simulink model "Nealinearni_realni_v2"  (R2023b)
settings: Solver=ode23t  StartTime=0.0  StopTime=stepp.sim_time  RelTol=1e-3
undefined symbols (not defined in the file or in its folder): boost, ccm_m_op, Ci, dcm_op, dcm_separate_tfs, G_sys_ccm, Ipv0, m0_ccm, pv, Ramp, Ru, sim_op, stepp
libraries: spsSeriesRLCBranchLib x6, spsCurrentMeasurementLib x3, spsVoltageMeasurementLib x3, spsBistableLib x2, dspstat3 x2, dspfdesign x1, spsDiodeLib x1, spsControlledCurrentSourceLib x1, spsIdealSwitchLib x1, simulink_extras x1, simulink x1, sps_lib x1
settings Model: Creator=teo  LastModifiedBy=teo
settings HardwareCC: ProdBitPerLong=64  ProdHWDeviceType=AMD->x86-64 (Linux 64)

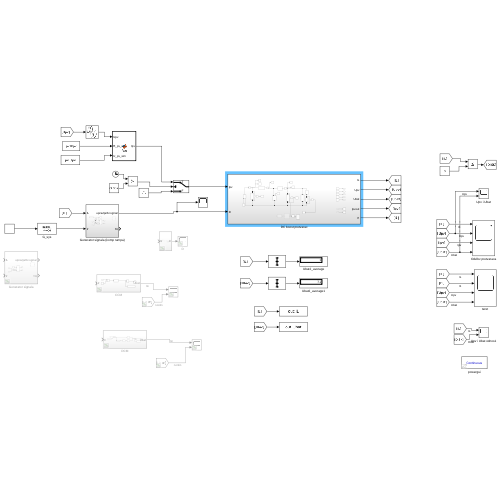
[thumbnail: Simulink's stored preview of the top-level diagram]
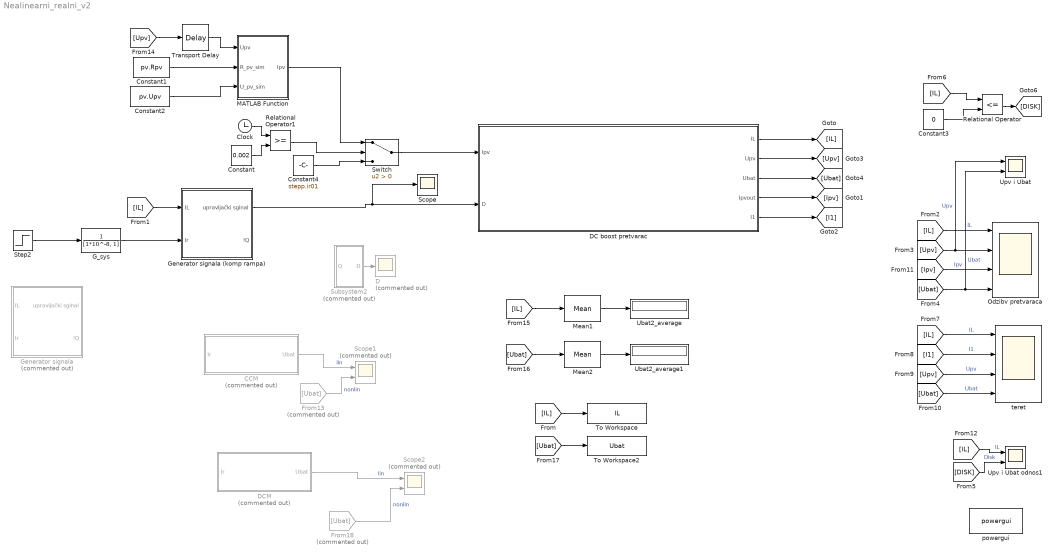
== system Nealinearni_realni_v2 ==
  CCM : Subsystem  Commented=on
  Clock : Clock
  Constant : Constant  Value=0.002
  Constant1 : Constant  Value=pv.Rpv
  Constant2 : Constant  Value=pv.Upv
  Constant3 : Constant  Value=0
  Constant4 : Constant  Value=stepp.ir01
  D : Scope  Commented=on
  DC boost pretvarac : Subsystem
  DCM : Subsystem  Commented=on
  From13 : From  Commented=on  GotoTag=Ubat
  From18 : From  Commented=on  GotoTag=Ubat
  G_sys : TransferFcn  Numerator=1  Denominator=[1*10^-8, 1]
  Generator signala : Subsystem  Commented=on
  Generator signala (komp rampa) : Subsystem
  MATLAB Function : MATLAB Function  TreatAsAtomicUnit=on
  Mean1 : dspstat3/Mean  run=off  InputProcessing=Columns as channels (frame based)  reset_popup=None  directionMode=Entire input  dimension=1  roiEnable=off  roiType=Rectangles  roiPortion=Entire ROI  roiOutput=Individual statistics for each ROI  roiFlag=off  roundingMode=Floor  overflowMode=off  outputDataTypeStr=Inherit: Same as accumulator  outputMin=[]  outputMax=[]  outputLastDataTypeStr=Inherit: Same as accumulator
  Mean2 : dspstat3/Mean  run=off  InputProcessing=Columns as channels (frame based)  reset_popup=None  directionMode=Entire input  dimension=1  roiEnable=off  roiType=Rectangles  roiPortion=Entire ROI  roiOutput=Individual statistics for each ROI  roiFlag=off  roundingMode=Floor  overflowMode=off  outputDataTypeStr=Inherit: Same as accumulator  outputMin=[]  outputMax=[]  outputLastDataTypeStr=Inherit: Same as accumulator
  Odzibv pretvaraca : Scope  NumInputPorts=4
  Relational Operator : RelationalOperator  Operator=<=  OutDataTypeStr=boolean  RndMeth=Simplest  InputSameDT=off
  Relational Operator1 : RelationalOperator  OutDataTypeStr=boolean  RndMeth=Simplest  InputSameDT=off
  Scope : Scope
  Scope1 : Scope  Commented=on  NumInputPorts=2
  Scope2 : Scope  Commented=on  NumInputPorts=2
  Step2 : Step  Time=stepp.step_time  Before=stepp.ir01  After=stepp.ir02  SampleTime=0
  Subsystem2 : Subsystem  Commented=on
  Switch : Switch  Criteria=u2 > Threshold  SaturateOnIntegerOverflow=off  InputSameDT=off
  To Workspace : ToWorkspace  VariableName=IL  SaveFormat=Timeseries  SampleTime=1e-6
  To Workspace2 : ToWorkspace  VariableName=Ubat  SaveFormat=Timeseries  SampleTime=1e-6
  Transport Delay : TransportDelay  DelayTime=0.001  BufferSize=4024
  Ubat2_average : Display
  Ubat2_average1 : Display
  Upv i Ubat : Scope  NumInputPorts=2
  Upv i Ubat odnos1 : Scope  NumInputPorts=2
  powergui : sps_lib/powergui  Priority=1  SimulationMode=Continuous  SampleTime=50e-6  frequency=60  Iterations=50  frequencyindice=0  Pbase=100e6  ErrMax=1e-4  UnitsV=kV  UnitsW=MW  buscounter=0  FunctionMessages=off  echomessages=off  EnableUseOfTLC=off  CurrentSourceSwitches=off  DisableSnubberDevices=off  DisableRonSwitches=off  DisableVfSwitches=off  DisplayEquations=off  AutomaticDiscreteSolvers=off  SolverType=Tustin/Backward Euler (TBE)  Interpol=off  ExternalGateDelay=off  methode=off  Ts=100  x0status=blocks  SPID=on  SwTol=0  HookPort=off  NonlinearTolerance=1e-4  nMaxIteration=100  ContinueOnMaxIteration=off  RestoreLinks=warning  ResistiveCurrentMeasurement=off  Frange=[0:2:500]  Ylog=off  Xlog=on  ShowGrid=off  save=off  variable=ZData  structure=0  ZoomFFT=off  StartTime=0.0  cycles=1  DisplayStyle=1  fundamental=60  FreqAxis=off  MaxFrequency=1000  frequencyindicesteady=1  RmsSteady=1  display=off
  teret : Scope  NumInputPorts=4
  wires:
  [IL] -> Odzibv pretvaraca/1  "IL"
  [Upv] -> Upv i Ubat/1, Odzibv pretvaraca/2  "Upv"
  [IL] -> teret/1  "IL"
  [I1] -> teret/2  "I1"
  [Upv] -> teret/3  "Upv"
  [IL] -> Upv i Ubat odnos1/1  "IL"
  [DISK] -> Upv i Ubat odnos1/2  "Disk"
  [Ipv] -> Odzibv pretvaraca/3  "Ipv"
  [IL] -> Relational Operator/1
  Relational Operator/1 -> [DISK]
  Constant3/1 -> Relational Operator/2
  [Ubat] -> Upv i Ubat/2, Odzibv pretvaraca/4  "Ubat"
  [Ubat] -> teret/4  "Ubat"
  DC boost pretvarac/2(Upv) -> [Upv]
  DC boost pretvarac/1(IL) -> [IL]
  DC boost pretvarac/3(Ubat) -> [Ubat]
  DC boost pretvarac/4(Ipvout) -> [Ipv]
  DC boost pretvarac/5(I1) -> [I1]
  [IL] -> Mean1/1
  Mean1/1 -> Ubat2_average/1
  [Ubat] -> Mean2/1
  Mean2/1 -> Ubat2_average1/1
  [IL] -> To Workspace/1
  [Ubat] -> To Workspace2/1
  Subsystem2/1(D) -> D/1
  Constant1/1 -> MATLAB Function/2(R_pv_sim)
  Constant2/1 -> MATLAB Function/3(U_pv_sim)
  [Upv] -> Transport Delay/1
  Transport Delay/1 -> MATLAB Function/1(Upv)
  Switch/1 -> DC boost pretvarac/1(Ipv)
  Clock/1 -> Relational Operator1/1
  Constant/1 -> Relational Operator1/2
  Relational Operator1/1 -> Switch/2
  Constant4/1 -> Switch/3
  MATLAB Function/1(Ipv) -> Switch/1
  CCM/1(Ubat) -> Scope1/1  "lin"
  From13/1 -> Scope1/2  "nonlin"
  DCM/1(Ubat) -> Scope2/1  "lin"
  From18/1 -> Scope2/2  "nonlin"
  [IL] -> Generator signala (komp rampa)/1(IL)
  Generator signala (komp rampa)/1(upravljački sginal) -> Scope/1, DC boost pretvarac/2(D)
  Step2/1 -> G_sys/1
  G_sys/1 -> Generator signala (komp rampa)/2(Ir)

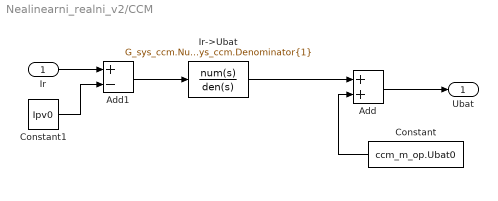
== system Nealinearni_realni_v2/CCM ==
  Ir : Inport
  Add : Sum
  Add1 : Sum  Inputs=+-
  Constant : Constant  Value=ccm_m_op.Ubat0
  Constant1 : Constant  Value=Ipv0
  Ir->Ubat : TransferFcn  Numerator=G_sys_ccm.Numerator{1}  Denominator=G_sys_ccm.Denominator{1}
  Ubat : Outport
  wires:
  Ir/1 -> Add1/1
  Constant1/1 -> Add1/2
  Add1/1 -> Ir->Ubat/1
  Add/1 -> Ubat/1
  Constant/1 -> Add/2
  Ir->Ubat/1 -> Add/1

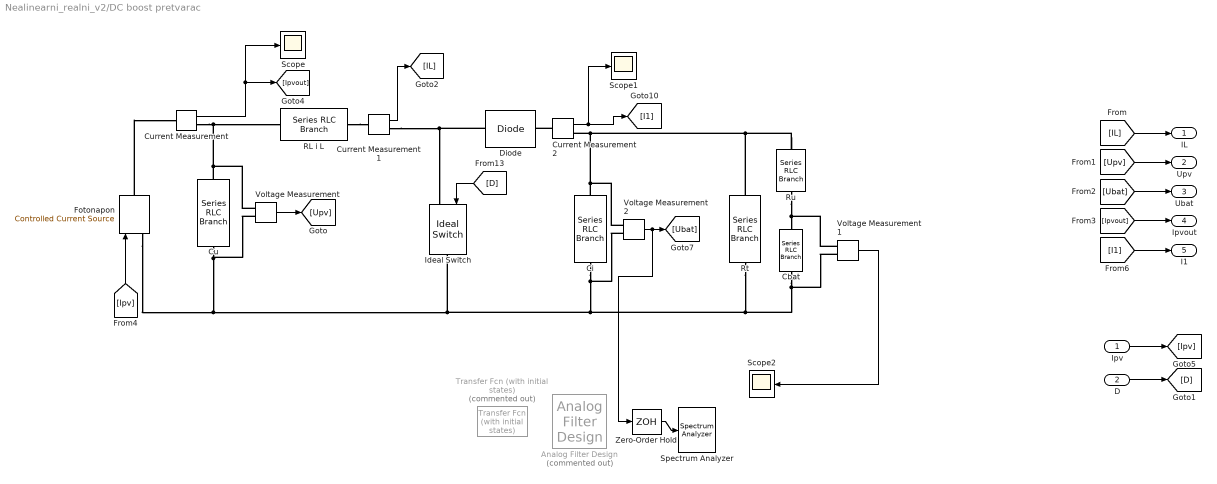
== system Nealinearni_realni_v2/DC boost pretvarac ==
  Ipv : Inport
  D : Inport  Port=2
  Analog Filter Design : dspfdesign/Analog Filter Design  Commented=on  method=Elliptic  filttype=Lowpass  N=8  Wlo=2*pi*boost.f  Whi=80  Rp=1  Rs=100
  Cbat : spsSeriesRLCBranchLib/Series RLC Branch  LConnTagsString=__new0  RConnTagsString=__new0  BranchType=C  Resistance=Ru  Inductance=1e-3  SetiL0=off  InitialCurrent=0  Capacitance=boost.Cbat  Setx0=on  InitialVoltage=sim_op.Ubat0  Measurements=None
  Ci : spsSeriesRLCBranchLib/Series RLC Branch  LConnTagsString=__new0  RConnTagsString=__new0  BranchType=C  Resistance=0.001  Inductance=1e-3  SetiL0=off  InitialCurrent=0  Capacitance=boost.Ci  Setx0=on  InitialVoltage=dcm_op.Ubat0  Measurements=None
  Cu : spsSeriesRLCBranchLib/Series RLC Branch  LConnTagsString=__new0  RConnTagsString=__new0  BranchType=C  Resistance=0.001  Inductance=1e-3  SetiL0=off  InitialCurrent=0  Capacitance=boost.Cu  Setx0=on  InitialVoltage=sim_op.Upv0  Measurements=None
  Current Measurement : spsCurrentMeasurementLib/Current Measurement  PhasorSimulation=off  OutputType=Complex  PSBequivalent=0
  Current Measurement1 : spsCurrentMeasurementLib/Current Measurement  PhasorSimulation=off  OutputType=Complex  PSBequivalent=0
  Current Measurement2 : spsCurrentMeasurementLib/Current Measurement  PhasorSimulation=off  OutputType=Complex  PSBequivalent=0
  Diode : spsDiodeLib/Diode  Ron=0  Lon=0  Vf=0  IC=0  UseSnubber=0  Rs=0  Cs=0  Measurements=off
  Fotonapon : spsControlledCurrentSourceLib/Controlled Current Source  Initialize=on  Source_Type=DC  Amplitude=0  Phase=0  Frequency=0  Measurements=None
  Ideal Switch : spsIdealSwitchLib/Ideal Switch  Ron=0  Lon=0  IC=0  Rs=0  Cs=0  Measurements=off
  RL i L : spsSeriesRLCBranchLib/Series RLC Branch  LConnTagsString=__new0  RConnTagsString=__new0  BranchType=RL  Resistance=boost.RL  Inductance=boost.L  SetiL0=off  InitialCurrent=Ipv0  Capacitance=1e-6  Setx0=off  InitialVoltage=0  Measurements=None
  Rt : spsSeriesRLCBranchLib/Series RLC Branch  LConnTagsString=__new0  RConnTagsString=__new0  BranchType=R  Resistance=boost.Rt  Inductance=1e-3  SetiL0=off  InitialCurrent=0  Capacitance=Ci  Setx0=off  InitialVoltage=0  Measurements=None
  Ru : spsSeriesRLCBranchLib/Series RLC Branch  LConnTagsString=__new0  RConnTagsString=__new0  BranchType=R  Resistance=boost.Ru  Inductance=1e-3  SetiL0=off  InitialCurrent=0  Capacitance=Ci  Setx0=on  InitialVoltage=Ubat0_ccm  Measurements=None
  Scope : Scope
  Scope1 : Scope
  Scope2 : Scope
  Spectrum Analyzer : SpectrumAnalyzer  WindowPosition=[1.000000,1.000000,1920.000000,1048.000000,]  Visible=on  ScopeFrameLocation=window  Method=Welch  PlotAsTwoSidedSpectrum=off  Span=150000  CenterFrequency=75000  StartFrequency=0  StopFrequency=150000  AveragingMethod=Exponential  ForgettingFactor=1  YLimits=[-161.71301101,85.74204889]  ExpandToolstrip=on  SelectedToolstripTab=spectrumAnalyzerToolstrip.measurementsTab
  Transfer Fcn (with initial states) : simulink_extras/Additional Linear/Transfer Fcn (with initial states)  Commented=on  N=[1]  D=[boost.Tmfc, 1]  X0=.5
  Voltage Measurement : spsVoltageMeasurementLib/Voltage Measurement  PhasorSimulation=off  OutputType=Complex  PSBequivalent=0
  Voltage Measurement1 : spsVoltageMeasurementLib/Voltage Measurement  PhasorSimulation=off  OutputType=Complex  PSBequivalent=0
  Voltage Measurement2 : spsVoltageMeasurementLib/Voltage Measurement  PhasorSimulation=off  OutputType=Complex  PSBequivalent=0
  Zero-Order Hold : ZeroOrderHold  SampleTime=1/(3*boost.f)
  IL : Outport
  Upv : Outport  Port=2
  Ubat : Outport  Port=3
  Ipvout : Outport  Port=4
  I1 : Outport  Port=5
  wires:
  Current Measurement1/1 -> [IL]
  Voltage Measurement/1 -> [Upv]
  [D] -> Ideal Switch/1
  [Ipv] -> Fotonapon/1
  D/1 -> [D]
  Ipv/1 -> [Ipv]
  [IL] -> IL/1
  [Upv] -> Upv/1
  [Ubat] -> Ubat/1
  Current Measurement/1 -> Scope/1, [Ipvout]
  [Ipvout] -> Ipvout/1
  Current Measurement2/1 -> Scope1/1, [I1]
  [I1] -> I1/1
  Voltage Measurement2/1 -> Zero-Order Hold/1, [Ubat]
  Voltage Measurement1/1 -> Scope2/1
  Zero-Order Hold/1 -> Spectrum Analyzer/1
  connections:
  Current Measurement/RConn1 -- Voltage Measurement/LConn1 -- Cu/LConn1 -- RL i L/LConn1
  RL i L/RConn1 -- Current Measurement1/LConn1
  Diode/LConn1 -- Ideal Switch/LConn1 -- Current Measurement1/RConn1
  Current Measurement2/LConn1 -- Diode/RConn1
  Ci/RConn1 -- Voltage Measurement2/LConn2 -- Voltage Measurement1/LConn2 -- Cbat/RConn1 -- Rt/RConn1 -- Voltage Measurement/LConn2 -- Cu/RConn1 -- Fotonapon/LConn1 -- Ideal Switch/RConn1
  Fotonapon/RConn1 -- Current Measurement/LConn1
  Ci/LConn1 -- Voltage Measurement2/LConn1 -- Rt/LConn1 -- Ru/LConn1 -- Current Measurement2/RConn1
  Ru/RConn1 -- Voltage Measurement1/LConn1 -- Cbat/LConn1

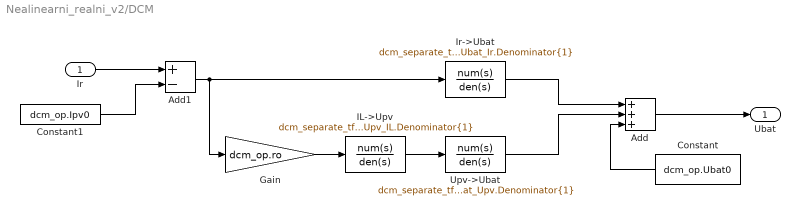
== system Nealinearni_realni_v2/DCM ==
  Ir : Inport
  Add : Sum  Inputs=+++
  Add1 : Sum  Inputs=+-
  Constant : Constant  Value=dcm_op.Ubat0
  Constant1 : Constant  Value=dcm_op.Ipv0
  Gain : Gain  Gain=dcm_op.ro
  IL->Upv : TransferFcn  Numerator=dcm_separate_tfs.G_Upv_IL.Numerator{1}  Denominator=dcm_separate_tfs.G_Upv_IL.Denominator{1}
  Ir->Ubat : TransferFcn  Numerator=dcm_separate_tfs.G_Ubat_Ir.Numerator{1}  Denominator=dcm_separate_tfs.G_Ubat_Ir.Denominator{1}
  Upv->Ubat : TransferFcn  Numerator=dcm_separate_tfs.G_Ubat_Upv.Numerator{1}  Denominator=dcm_separate_tfs.G_Ubat_Upv.Denominator{1}
  Ubat : Outport
  wires:
  Ir/1 -> Add1/1
  Add/1 -> Ubat/1
  Ir->Ubat/1 -> Add/1
  Constant1/1 -> Add1/2
  Upv->Ubat/1 -> Add/2
  Constant/1 -> Add/3
  IL->Upv/1 -> Upv->Ubat/1
  Add1/1 -> Gain/1, Ir->Ubat/1
  Gain/1 -> IL->Upv/1

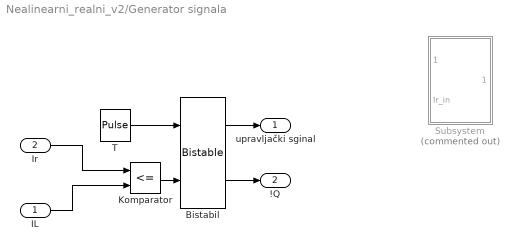
== system Nealinearni_realni_v2/Generator signala ==
  IL : Inport
  Ir : Inport  Port=2
  Bistabil : spsBistableLib/Bistable  Qpriority=Set  ic=0  Ts=0
      settings: LibrarySourceBlock=sps_lib/Control/Bistable
  Komparator : RelationalOperator  Operator=<=  OutDataTypeStr=boolean  RndMeth=Simplest  InputSameDT=off
  Subsystem : Subsystem  Commented=on
  T : DiscretePulseGenerator  PulseType=Time based  Period=boost.T
  upravljački sginal : Outport
  !Q : Outport  Port=2
  wires:
  Komparator/1 -> Bistabil/2
  Bistabil/2 -> !Q/1
  Bistabil/1 -> upravljački sginal/1
  IL/1 -> Komparator/2
  T/1 -> Bistabil/1
  Ir/1 -> Komparator/1

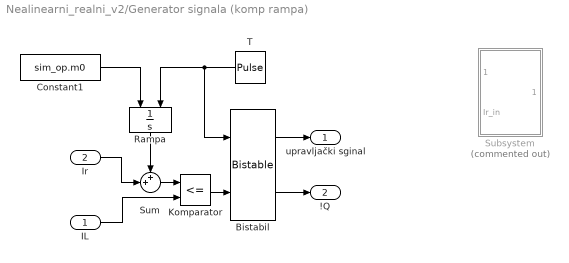
== system Nealinearni_realni_v2/Generator signala (komp rampa) ==
  IL : Inport
  Ir : Inport  Port=2
  Bistabil : spsBistableLib/Bistable  Qpriority=Set  ic=0  Ts=0
      settings: LibrarySourceBlock=sps_lib/Control/Bistable
  Constant1 : Constant  Value=sim_op.m0
  Komparator : RelationalOperator  Operator=<=  OutDataTypeStr=boolean  RndMeth=Simplest  InputSameDT=off
  Rampa : Integrator  ExternalReset=rising
  Subsystem : Subsystem  Commented=on
  Sum : Sum  Inputs=++|
  T : DiscretePulseGenerator  PulseType=Time based  Period=boost.T
  upravljački sginal : Outport
  !Q : Outport  Port=2
  wires:
  Komparator/1 -> Bistabil/2
  Bistabil/2 -> !Q/1
  Bistabil/1 -> upravljački sginal/1
  IL/1 -> Komparator/2
  Sum/1 -> Komparator/1
  Ir/1 -> Sum/2
  Rampa/1 -> Sum/1
  T/1 -> Bistabil/1, Rampa/2
  Constant1/1 -> Rampa/1

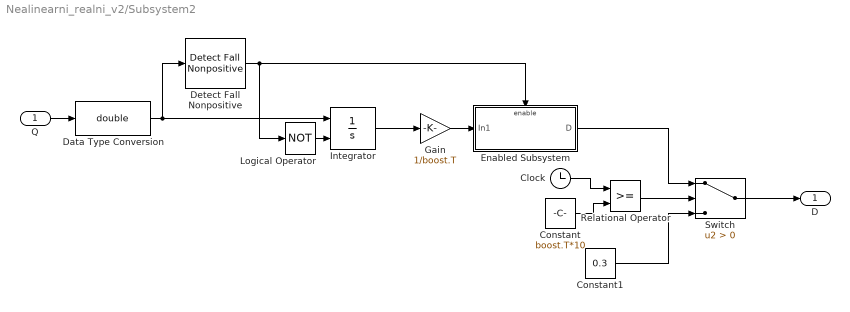
== system Nealinearni_realni_v2/Subsystem2 ==
  Q : Inport
  Clock : Clock
  Constant : Constant  Value=boost.T*10
  Constant1 : Constant  Value=0.3
  Data Type Conversion : DataTypeConversion  OutDataTypeStr=double  SaturateOnIntegerOverflow=off  RndMeth=Floor
  Detect Fall Nonpositive : simulink/Logic and Bit Operations/Detect Fall Nonpositive  vinit=0  OutDataTypeStr=boolean
  Enabled Subsystem : Subsystem  TreatAsAtomicUnit=on
  Gain : Gain  Gain=1/boost.T
  Integrator : Integrator  ExternalReset=rising
  Logical Operator : Logic  Operator=NOT  AllPortsSameDT=off  OutDataTypeStr=boolean
  Relational Operator : RelationalOperator  OutDataTypeStr=boolean  RndMeth=Simplest  InputSameDT=off
  Switch : Switch  Criteria=u2 > Threshold  SaturateOnIntegerOverflow=off  InputSameDT=off
  D : Outport
  wires:
  Integrator/1 -> Gain/1
  Gain/1 -> Enabled Subsystem/1(In1)
  Enabled Subsystem/1(D) -> Switch/1
  Switch/1 -> D/1
  Clock/1 -> Relational Operator/1
  Constant/1 -> Relational Operator/2
  Relational Operator/1 -> Switch/2
  Constant1/1 -> Switch/3
  Q/1 -> Data Type Conversion/1
  Data Type Conversion/1 -> Detect Fall Nonpositive/1, Integrator/1
  Logical Operator/1 -> Integrator/2
  Detect Fall Nonpositive/1 -> Logical Operator/1, Enabled Subsystem/Enable

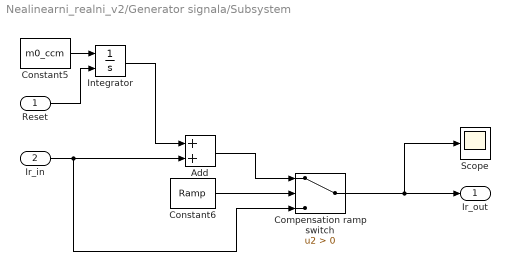
== system Nealinearni_realni_v2/Generator signala/Subsystem ==
  Reset : Inport
  Ir_in : Inport  Port=2
  Add : Sum
  Compensation ramp switch : Switch  Criteria=u2 > Threshold  SaturateOnIntegerOverflow=off  InputSameDT=off
  Constant5 : Constant  Value=m0_ccm
  Constant6 : Constant  Value=Ramp
  Integrator : Integrator  ExternalReset=rising
  Scope : Scope
  Ir_out : Outport
  wires:
  Constant5/1 -> Integrator/1
  Integrator/1 -> Add/1
  Add/1 -> Compensation ramp switch/1
  Reset/1 -> Integrator/2
  Compensation ramp switch/1 -> Scope/1, Ir_out/1
  Constant6/1 -> Compensation ramp switch/2
  Ir_in/1 -> Compensation ramp switch/3, Add/2

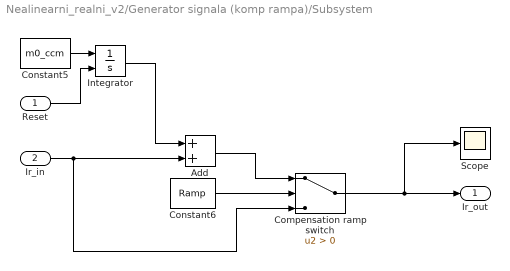
== system Nealinearni_realni_v2/Generator signala (komp rampa)/Subsystem ==
  Reset : Inport
  Ir_in : Inport  Port=2
  Add : Sum
  Compensation ramp switch : Switch  Criteria=u2 > Threshold  SaturateOnIntegerOverflow=off  InputSameDT=off
  Constant5 : Constant  Value=m0_ccm
  Constant6 : Constant  Value=Ramp
  Integrator : Integrator  ExternalReset=rising
  Scope : Scope
  Ir_out : Outport
  wires:
  Constant5/1 -> Integrator/1
  Integrator/1 -> Add/1
  Add/1 -> Compensation ramp switch/1
  Reset/1 -> Integrator/2
  Compensation ramp switch/1 -> Scope/1, Ir_out/1
  Constant6/1 -> Compensation ramp switch/2
  Ir_in/1 -> Compensation ramp switch/3, Add/2

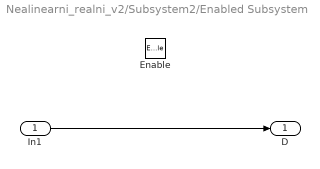
== system Nealinearni_realni_v2/Subsystem2/Enabled Subsystem ==
  In1 : Inport
  Enable : EnablePort
  D : Outport
  wires:
  In1/1 -> D/1

== matlab function Nealinearni_realni_v2/MATLAB Function ==
  data: Upv input; Ipv output; R_pv_sim input; U_pv_sim input
function Ipv = fcn(Upv, R_pv_sim, U_pv_sim)

R = interp1(U_pv_sim, R_pv_sim, Upv, 'linear', 'extrap');

Ipv = Upv/R;
